simulink library "triad_coarse_estimator"  (R2016b)
settings: Solver=VariableStepAuto  StartTime=0.0  StopTime=10.0  RelTol=1e-3
undefined symbols (not defined in the file): fsw_params
libraries: dspmathops x6, vrlib x4
settings Model: Creator=sexymathemagician  LastModifiedBy=Taylor

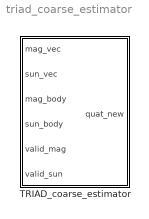
== system triad_coarse_estimator ==
  TRIAD_coarse_estimator : Subsystem

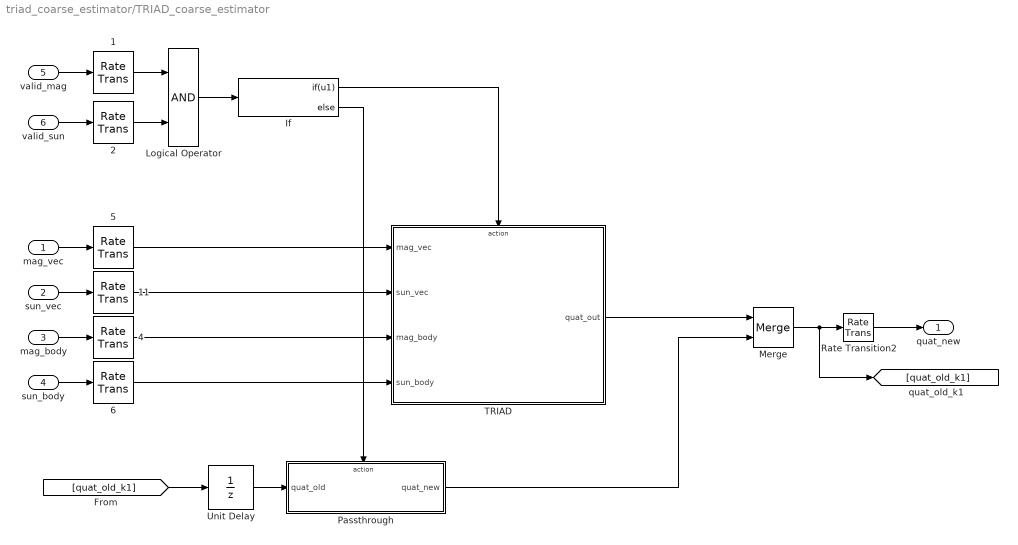
== system triad_coarse_estimator/TRIAD_coarse_estimator ==
  "mag_vec " : Inport
  "sun_vec " : Inport  Port=2
  mag_body : Inport  Port=3
  sun_body : Inport  Port=4
  valid_mag : Inport  Port=5
  valid_sun : Inport  Port=6
  " 1" : RateTransition  X0=fsw_params.estimation.ic.rt_valid_mag  OutPortSampleTime=fsw_params.estimation.sample_time_s
  " 11" : RateTransition  X0=fsw_params.estimation.ic.rt_sun_eci_est  OutPortSampleTime=fsw_params.estimation.sample_time_s
  " 2" : RateTransition  X0=fsw_params.estimation.ic.rt_valid_sun  OutPortSampleTime=fsw_params.estimation.sample_time_s
  " 4" : RateTransition  X0=fsw_params.estimation.ic.rt_mag_body  OutPortSampleTime=fsw_params.estimation.sample_time_s
  " 5" : RateTransition  X0=fsw_params.estimation.ic.rt_mag_eci_est  OutPortSampleTime=fsw_params.estimation.sample_time_s
  " 6" : RateTransition  X0=fsw_params.estimation.ic.rt_sun_body  OutPortSampleTime=fsw_params.estimation.sample_time_s
  If : If  IfExpression=u1
  Logical Operator : Logic  AllPortsSameDT=off  OutDataTypeStr=boolean
  Merge : Merge
  Passthrough : Subsystem  TreatAsAtomicUnit=on
  Rate Transition2 : RateTransition  X0=fsw_params.estimation.ic.quat_est_init
  "TRIAD " : Subsystem  TreatAsAtomicUnit=on
  Unit Delay : UnitDelay  InitialCondition=fsw_params.estimation.ic.quat_est_init  SampleTime=fsw_params.estimation.sample_time_s
  quat_new : Outport
  wires:
  "mag_vec "/1 -> " 5"/1
  "sun_vec "/1 -> " 11"/1
  mag_body/1 -> " 4"/1
  sun_body/1 -> " 6"/1
  If/1 -> "TRIAD "/Action
  If/2 -> Passthrough/Action
  "TRIAD "/1("quat_out ") -> Merge/1
  Passthrough/1(quat_new) -> Merge/2
  Merge/1 -> [quat_old_k1], Rate Transition2/1
  valid_mag/1 -> " 1"/1
  valid_sun/1 -> " 2"/1
  Logical Operator/1 -> If/1
  Rate Transition2/1 -> quat_new/1
  " 1"/1 -> Logical Operator/1
  " 2"/1 -> Logical Operator/2
  " 4"/1 -> "TRIAD "/3(mag_body)
  " 6"/1 -> "TRIAD "/4(sun_body)
  " 11"/1 -> "TRIAD "/2("sun_vec ")
  " 5"/1 -> "TRIAD "/1("mag_vec ")
  [quat_old_k1] -> Unit Delay/1
  Unit Delay/1 -> Passthrough/1(quat_old)

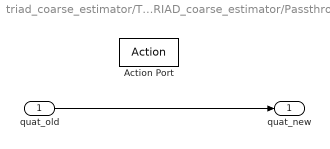
== system triad_coarse_estimator/TRIAD_coarse_estimator/Passthrough ==
  quat_old : Inport
  Action Port : ActionPort
  quat_new : Outport
  wires:
  quat_old/1 -> quat_new/1

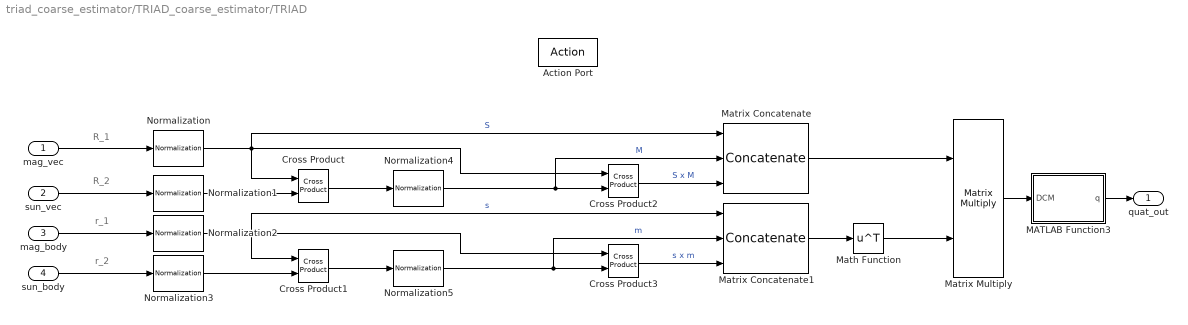
== system triad_coarse_estimator/TRIAD_coarse_estimator/TRIAD  ==
  note: R_2
  note: R_1
  note: r_2
  note: r_1
  "mag_vec " : Inport
  "sun_vec " : Inport  Port=2
  mag_body : Inport  Port=3
  sun_body : Inport  Port=4
  Action Port : ActionPort
  Cross Product{,1..3} (4 alike) : vrlib/Utilities/Cross Product
  MATLAB Function3 : MATLAB Function  TreatAsAtomicUnit=on
  Math Function : Math  Operator=transpose  SaturateOnIntegerOverflow=on
  Matrix Concatenate : Concatenate  NumInputs=3  Mode=Multidimensional array  ConcatenateDimension=2
  Matrix Concatenate1 : Concatenate  NumInputs=3  Mode=Multidimensional array  ConcatenateDimension=2
  Matrix Multiply : Product  Multiplication=Matrix(*)
  Normalization{,1..5} (6 alike) : dspmathops/Normalization  NormType=2-norm  Bias=1e-10  NormOver=Each column  Dimension=1  outputDataTypeStr=Inherit: Same as product output  outputLastDataTypeStr=Inherit: Same as product output  outputMin=[]  outputMax=[]  accumDataTypeStr=Inherit: Same as product output  accumLastDataTypeStr=Inherit: Same as product output  roundingMode=Floor  overflowMode=off
  "quat_out " : Outport
  wires:
  "mag_vec "/1 -> Normalization/1
  "sun_vec "/1 -> Normalization1/1
  mag_body/1 -> Normalization2/1
  sun_body/1 -> Normalization3/1
  Normalization1/1 -> Cross Product/2
  Normalization2/1 -> Matrix Concatenate1/1, Cross Product3/1, Cross Product1/1  "s"
  Normalization3/1 -> Cross Product1/2
  Cross Product/1 -> Normalization4/1
  Cross Product1/1 -> Normalization5/1
  Normalization4/1 -> Matrix Concatenate/2, Cross Product2/2  "M"
  Normalization5/1 -> Matrix Concatenate1/2, Cross Product3/2  "m"
  Cross Product2/1 -> Matrix Concatenate/3  "S x M"
  Cross Product3/1 -> Matrix Concatenate1/3  "s x m"
  Matrix Concatenate1/1 -> Math Function/1
  Matrix Concatenate/1 -> Matrix Multiply/1
  Math Function/1 -> Matrix Multiply/2
  MATLAB Function3/1(q) -> "quat_out "/1
  Matrix Multiply/1 -> MATLAB Function3/1(DCM)
  Normalization/1 -> Matrix Concatenate/1, Cross Product/1, Cross Product2/1  "S"

== matlab function triad_coarse_estimator/TRIAD_coarse_estimator/TRIAD /MATLAB Function3 ==
  data: DCM input; q output
function q = myDCM2quat( DCM )
% ----------------------------------------------------------------------- %
% UW HuskySat-1, ADCS Team
%
% DCM to Quaternion conversion assuming positive scalar part
%
% T. Reynolds 1.15.18
% #codegen
% ----------------------------------------------------------------------- %
q   = zeros(4,1);

tr  = trace(DCM);

q(1)    = 0.5*sqrt(tr + 1);

if( q(1) ~= 0 )
    eta     = 1/(4*q(1));
    q(2)    = eta*(DCM(2,3) - DCM(3,2));
    q(3)    = eta*(DCM(3,1) - DCM(1,3));
    q(4)    = eta*(DCM(1,2) - DCM(2,1));
else
    q(2)  = sqrt(0.5*(DCM(1,1) + 1));
    q(3)  = sign(DCM(1,2))*sqrt(0.5*(DCM(2,2) + 1));
    q(4)  = sign(DCM(1,3))*sqrt(0.5*(DCM(3,3) + 1));
end


end
